simulink model "flc_ann_master"  (R2025a)
settings: Solver=ode23tb  StartTime=0.0  StopTime=2  FixedStep=1e-8  MaxStep=1e-5  RelTol=1e-4
values from neighbouring files (symbols this model uses):
  init_duty = 0.5    [params.m]    (also in sim_duties.m = init_duty_array(i))
  irr_final_1 = 1000    [sim_duties.m]
  irr_final_2 = 1000    [sim_duties.m]
  irr_final_3 = 1000    [sim_duties.m]
  irr_final_4 = 1000    [sim_duties.m]
  irr_final_5 = 1000    [sim_duties.m]
  irr_init_1 = 1000    [sim_duties.m]
  irr_init_2 = 1000    [sim_duties.m]
  irr_init_3 = 1000    [sim_duties.m]
  irr_init_4 = 1000    [sim_duties.m]
  irr_init_5 = 1000    [sim_duties.m]
  sample_time_FLC = 0.005    [params.m]    (also in sim_duties.m)
  sample_time_mv_avg = 1e-4    (= 0.0001)    [params.m]    (also in sim_duties.m)
  temp = 25    [params.m]    (also in sim_duties.m)
undefined symbols (not defined in the file or in its folder): DiscIntNeverNeededParam, t_step
libraries: neural x36, spsMosfetLib x5, spsSeriesRLCBranchLib x5, eeGeneralControl x3, spsCurrentMeasurementLib x2, spsDiodeLib x2, spsFirstOrderFilterLib x2, slpidlib x2, simulink x2, spsVoltageMeasurementLib x2, spsACVoltageSourceLib x1, spsAlphaBetaZerotodq0Lib x1
(part 2 of 2)

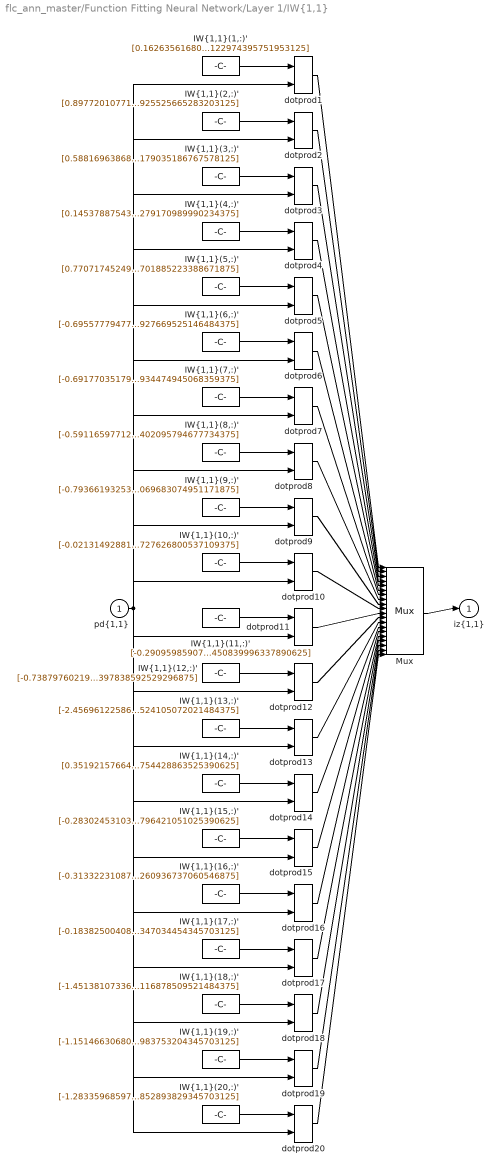
== system flc_ann_master/Function Fitting Neural Network/Layer 1/IW{1,1} ==
  "pd{1,1}" : Inport  PortDimensions=5
      mask Display: e = 0.06;c1 = [120 230 180]/255;c2 = ([120 230 180]+0)/(256+128);c3 = ([120 230 180]+128)/(256+128);patch([0 1 1 0],[0 0 1 1],c1);patch([0 1 1 1-e 1-e 0+e],[0 0 1 1-e 0+e 0+e],c2);patch([0 0 1 1-e 0+e 0+e],[0 1 1 1-e 1-e 0+e],c3);plot([0 1 1 0 0],[0 0 1 1 0]);
  "IW{1,1}(1,:)'" : Constant  Value=[0.1626356168023161130609111069134087301790714263916015625;1.014539472778073214698224546737037599086761474609375;1.99974778893698879045359717565588653087615966796875;0.2096339514215423971421614623977802693843841552734375;-5.6789966587194289360240873065777122974395751953125]
      mask Display: e = 0.06;c1 = [120 150 230]/255;c2 = ([120 150 230]+0)/383;c3 = ([120 150 230]+128)/383;patch([0 1 1 0],[0 0 1 1],c1);patch([0 1 1 1-e 1-e 0+e],[0 0 1 1-e 0+e 0+e],c2);patch([0 0 1 1-e 0+e 0+e],[0 1 1 1-e 1-e 0+e],c3);plot([0 1 1 0 0],[0 0 1 1 0]);disp('Weights');
  "IW{1,1}(10,:)'" : Constant  Value=[-0.0213149288150113642992256046682086889632046222686767578125;-0.568850920387156566704334181849844753742218017578125;1.371346571730940322453307089745067059993743896484375;1.577494106987263666752596691367216408252716064453125;-0.39484466016965702461760656660771928727626800537109375]
      mask Display: e = 0.06;c1 = [120 150 230]/255;c2 = ([120 150 230]+0)/383;c3 = ([120 150 230]+128)/383;patch([0 1 1 0],[0 0 1 1],c1);patch([0 1 1 1-e 1-e 0+e],[0 0 1 1-e 0+e 0+e],c2);patch([0 0 1 1-e 0+e 0+e],[0 1 1 1-e 1-e 0+e],c3);plot([0 1 1 0 0],[0 0 1 1 0]);disp('Weights');
  "IW{1,1}(11,:)'" : Constant  Value=[-0.29095985907524279934222022347967140376567840576171875;1.4011731136993168522764108274714089930057525634765625;1.1829639348115577046627322488347999751567840576171875;-5.07892395952207653664345343713648617267608642578125;2.99724620350438275551141487085260450839996337890625]
      mask Display: e = 0.06;c1 = [120 150 230]/255;c2 = ([120 150 230]+0)/383;c3 = ([120 150 230]+128)/383;patch([0 1 1 0],[0 0 1 1],c1);patch([0 1 1 1-e 1-e 0+e],[0 0 1 1-e 0+e 0+e],c2);patch([0 0 1 1-e 0+e 0+e],[0 1 1 1-e 1-e 0+e],c3);plot([0 1 1 0 0],[0 0 1 1 0]);disp('Weights');
  "IW{1,1}(12,:)'" : Constant  Value=[-0.7387976021984303809375660421210341155529022216796875;-1.0178618623283923749767154731671325862407684326171875;-0.1381009052088023880688893996193655766546726226806640625;0.59120561994734599498002580730826593935489654541015625;1.826460521302780914965069314348511397838592529296875]
      mask Display: e = 0.06;c1 = [120 150 230]/255;c2 = ([120 150 230]+0)/383;c3 = ([120 150 230]+128)/383;patch([0 1 1 0],[0 0 1 1],c1);patch([0 1 1 1-e 1-e 0+e],[0 0 1 1-e 0+e 0+e],c2);patch([0 0 1 1-e 0+e 0+e],[0 1 1 1-e 1-e 0+e],c3);plot([0 1 1 0 0],[0 0 1 1 0]);disp('Weights');
  "IW{1,1}(13,:)'" : Constant  Value=[-2.456961225860202713278113151318393647670745849609375;-0.5049152215026426748778476394363678991794586181640625;0.3922518923682936087260486601735465228557586669921875;0.6442280759956335867144616713630966842174530029296875;-0.51190556258231667552394128506421111524105072021484375]
      mask Display: e = 0.06;c1 = [120 150 230]/255;c2 = ([120 150 230]+0)/383;c3 = ([120 150 230]+128)/383;patch([0 1 1 0],[0 0 1 1],c1);patch([0 1 1 1-e 1-e 0+e],[0 0 1 1-e 0+e 0+e],c2);patch([0 0 1 1-e 0+e 0+e],[0 1 1 1-e 1-e 0+e],c3);plot([0 1 1 0 0],[0 0 1 1 0]);disp('Weights');
  "IW{1,1}(14,:)'" : Constant  Value=[0.351921576647878431298721579878474585711956024169921875;-2.29066783338849599971354109584353864192962646484375;-1.1972818394599020752622209329274483025074005126953125;1.964498776969650695178870591917075216770172119140625;2.312458865409122044098921833210624754428863525390625]
      mask Display: e = 0.06;c1 = [120 150 230]/255;c2 = ([120 150 230]+0)/383;c3 = ([120 150 230]+128)/383;patch([0 1 1 0],[0 0 1 1],c1);patch([0 1 1 1-e 1-e 0+e],[0 0 1 1-e 0+e 0+e],c2);patch([0 0 1 1-e 0+e 0+e],[0 1 1 1-e 1-e 0+e],c3);plot([0 1 1 0 0],[0 0 1 1 0]);disp('Weights');
  "IW{1,1}(15,:)'" : Constant  Value=[-0.283024531034079596114594323807978071272373199462890625;-0.64693582354276502055512310107587836682796478271484375;-1.91800918516954066461721595260314643383026123046875;-2.092225653502387761051295456127263605594635009765625;1.516845141309114186611850527697242796421051025390625]
      mask Display: e = 0.06;c1 = [120 150 230]/255;c2 = ([120 150 230]+0)/383;c3 = ([120 150 230]+128)/383;patch([0 1 1 0],[0 0 1 1],c1);patch([0 1 1 1-e 1-e 0+e],[0 0 1 1-e 0+e 0+e],c2);patch([0 0 1 1-e 0+e 0+e],[0 1 1 1-e 1-e 0+e],c3);plot([0 1 1 0 0],[0 0 1 1 0]);disp('Weights');
  "IW{1,1}(16,:)'" : Constant  Value=[-0.313322310879322218912790276590385474264621734619140625;2.774701737691696035170707546058110892772674560546875;-4.53633611923154145273429094231687486171722412109375;-0.65501382413655140357633399617043323814868927001953125;-0.9854404943783190429229534856858663260936737060546875]
      mask Display: e = 0.06;c1 = [120 150 230]/255;c2 = ([120 150 230]+0)/383;c3 = ([120 150 230]+128)/383;patch([0 1 1 0],[0 0 1 1],c1);patch([0 1 1 1-e 1-e 0+e],[0 0 1 1-e 0+e 0+e],c2);patch([0 0 1 1-e 0+e 0+e],[0 1 1 1-e 1-e 0+e],c3);plot([0 1 1 0 0],[0 0 1 1 0]);disp('Weights');
  "IW{1,1}(17,:)'" : Constant  Value=[-0.1838250040857035416674847283502458594739437103271484375;1.130320574163679037127394622075371444225311279296875;-1.213329860734431608904060340137220919132232666015625;-1.884962772921485285593234948464669287204742431640625;0.98188732582681570448812635731883347034454345703125]
      mask Display: e = 0.06;c1 = [120 150 230]/255;c2 = ([120 150 230]+0)/383;c3 = ([120 150 230]+128)/383;patch([0 1 1 0],[0 0 1 1],c1);patch([0 1 1 1-e 1-e 0+e],[0 0 1 1-e 0+e 0+e],c2);patch([0 0 1 1-e 0+e 0+e],[0 1 1 1-e 1-e 0+e],c3);plot([0 1 1 0 0],[0 0 1 1 0]);disp('Weights');
  "IW{1,1}(18,:)'" : Constant  Value=[-1.4513810733606338221335363414254970848560333251953125;2.008917038973344393326669887755997478961944580078125;1.3543511781589836484585021025850437581539154052734375;0.07174802344186757829813672060481621883809566497802734375;0.28193094730051215801580610786913894116878509521484375]
      mask Display: e = 0.06;c1 = [120 150 230]/255;c2 = ([120 150 230]+0)/383;c3 = ([120 150 230]+128)/383;patch([0 1 1 0],[0 0 1 1],c1);patch([0 1 1 1-e 1-e 0+e],[0 0 1 1-e 0+e 0+e],c2);patch([0 0 1 1-e 0+e 0+e],[0 1 1 1-e 1-e 0+e],c3);plot([0 1 1 0 0],[0 0 1 1 0]);disp('Weights');
  "IW{1,1}(19,:)'" : Constant  Value=[-1.1514663068085624342273831643979065120220184326171875;1.380766100437355259344940350274555385112762451171875;-0.448457718469357835555655356074566952884197235107421875;1.169745525191284940547120640985667705535888671875;1.352602327310475249788623841595835983753204345703125]
      mask Display: e = 0.06;c1 = [120 150 230]/255;c2 = ([120 150 230]+0)/383;c3 = ([120 150 230]+128)/383;patch([0 1 1 0],[0 0 1 1],c1);patch([0 1 1 1-e 1-e 0+e],[0 0 1 1-e 0+e 0+e],c2);patch([0 0 1 1-e 0+e 0+e],[0 1 1 1-e 1-e 0+e],c3);plot([0 1 1 0 0],[0 0 1 1 0]);disp('Weights');
  "IW{1,1}(2,:)'" : Constant  Value=[0.897720107718310789124416260165162384510040283203125;0.6045958291500983516897349545615725219249725341796875;1.7980406071958838776225775291095487773418426513671875;-4.24893179252118624589229511911980807781219482421875;-0.7416107529120250507759237734717316925525665283203125]
      mask Display: e = 0.06;c1 = [120 150 230]/255;c2 = ([120 150 230]+0)/383;c3 = ([120 150 230]+128)/383;patch([0 1 1 0],[0 0 1 1],c1);patch([0 1 1 1-e 1-e 0+e],[0 0 1 1-e 0+e 0+e],c2);patch([0 0 1 1-e 0+e 0+e],[0 1 1 1-e 1-e 0+e],c3);plot([0 1 1 0 0],[0 0 1 1 0]);disp('Weights');
  "IW{1,1}(20,:)'" : Constant  Value=[-1.28335968597945448976815896457992494106292724609375;-1.4230720872940150201202413882128894329071044921875;-1.383852677357449767470143342507071793079376220703125;-0.2359179865147377486156443637810298241674900054931640625;-0.201423945604798593222994895768351852893829345703125]
      mask Display: e = 0.06;c1 = [120 150 230]/255;c2 = ([120 150 230]+0)/383;c3 = ([120 150 230]+128)/383;patch([0 1 1 0],[0 0 1 1],c1);patch([0 1 1 1-e 1-e 0+e],[0 0 1 1-e 0+e 0+e],c2);patch([0 0 1 1-e 0+e 0+e],[0 1 1 1-e 1-e 0+e],c3);plot([0 1 1 0 0],[0 0 1 1 0]);disp('Weights');
  "IW{1,1}(3,:)'" : Constant  Value=[0.5881696386836756662574998699710704386234283447265625;-0.89580513472184242207418947145924903452396392822265625;-1.5454054003772699221741504516103304922580718994140625;0.955378626380716244881341481232084333896636962890625;1.1847012618567938080360590902273543179035186767578125]
      mask Display: e = 0.06;c1 = [120 150 230]/255;c2 = ([120 150 230]+0)/383;c3 = ([120 150 230]+128)/383;patch([0 1 1 0],[0 0 1 1],c1);patch([0 1 1 1-e 1-e 0+e],[0 0 1 1-e 0+e 0+e],c2);patch([0 0 1 1-e 0+e 0+e],[0 1 1 1-e 1-e 0+e],c3);plot([0 1 1 0 0],[0 0 1 1 0]);disp('Weights');
  "IW{1,1}(4,:)'" : Constant  Value=[0.1453788754354973511428994470406905747950077056884765625;1.6569375264883834386608896238612942397594451904296875;-3.56372497066039262136882825870998203754425048828125;-0.8353641157188942401035092188976705074310302734375;1.2124796973580609371623495462699793279170989990234375]
      mask Display: e = 0.06;c1 = [120 150 230]/255;c2 = ([120 150 230]+0)/383;c3 = ([120 150 230]+128)/383;patch([0 1 1 0],[0 0 1 1],c1);patch([0 1 1 1-e 1-e 0+e],[0 0 1 1-e 0+e 0+e],c2);patch([0 0 1 1-e 0+e 0+e],[0 1 1 1-e 1-e 0+e],c3);plot([0 1 1 0 0],[0 0 1 1 0]);disp('Weights');
  "IW{1,1}(5,:)'" : Constant  Value=[0.77071745249031808899786710753687657415866851806640625;0.3806567747078062335930326298694126307964324951171875;-1.1569156708901997543392781153670512139797210693359375;3.0882529402780907190617654123343527317047119140625;-0.462094404994892016258489775282214395701885223388671875]
      mask Display: e = 0.06;c1 = [120 150 230]/255;c2 = ([120 150 230]+0)/383;c3 = ([120 150 230]+128)/383;patch([0 1 1 0],[0 0 1 1],c1);patch([0 1 1 1-e 1-e 0+e],[0 0 1 1-e 0+e 0+e],c2);patch([0 0 1 1-e 0+e 0+e],[0 1 1 1-e 1-e 0+e],c3);plot([0 1 1 0 0],[0 0 1 1 0]);disp('Weights');
  "IW{1,1}(6,:)'" : Constant  Value=[-0.695577794775811497629547375254333019256591796875;-1.701146701078736445111871944391168653964996337890625;-2.050427426016556697874193559982813894748687744140625;1.811004933153217422159286797977983951568603515625;-0.49416975187174771999565336955129168927669525146484375]
      mask Display: e = 0.06;c1 = [120 150 230]/255;c2 = ([120 150 230]+0)/383;c3 = ([120 150 230]+128)/383;patch([0 1 1 0],[0 0 1 1],c1);patch([0 1 1 1-e 1-e 0+e],[0 0 1 1-e 0+e 0+e],c2);patch([0 0 1 1-e 0+e 0+e],[0 1 1 1-e 1-e 0+e],c3);plot([0 1 1 0 0],[0 0 1 1 0]);disp('Weights');
  "IW{1,1}(7,:)'" : Constant  Value=[-0.69177035179182977397971399113885127007961273193359375;-0.205470533347971773263651584784383885562419891357421875;1.7003040131834559200996181971277110278606414794921875;2.216435685343544292891238001175224781036376953125;1.451900915541782577378171481541357934474945068359375]
      mask Display: e = 0.06;c1 = [120 150 230]/255;c2 = ([120 150 230]+0)/383;c3 = ([120 150 230]+128)/383;patch([0 1 1 0],[0 0 1 1],c1);patch([0 1 1 1-e 1-e 0+e],[0 0 1 1-e 0+e 0+e],c2);patch([0 0 1 1-e 0+e 0+e],[0 1 1 1-e 1-e 0+e],c3);plot([0 1 1 0 0],[0 0 1 1 0]);disp('Weights');
  "IW{1,1}(8,:)'" : Constant  Value=[-0.5911659771272115282414461034932173788547515869140625;0.9796323024744155727461247806786559522151947021484375;-0.51058490400159783906275379194994457066059112548828125;1.178946871689596331833627118612639605998992919921875;1.0642800652213446621630055233254097402095794677734375]
      mask Display: e = 0.06;c1 = [120 150 230]/255;c2 = ([120 150 230]+0)/383;c3 = ([120 150 230]+128)/383;patch([0 1 1 0],[0 0 1 1],c1);patch([0 1 1 1-e 1-e 0+e],[0 0 1 1-e 0+e 0+e],c2);patch([0 0 1 1-e 0+e 0+e],[0 1 1 1-e 1-e 0+e],c3);plot([0 1 1 0 0],[0 0 1 1 0]);disp('Weights');
  "IW{1,1}(9,:)'" : Constant  Value=[-0.79366193253040240307427666266448795795440673828125;-2.096544268041097947019579805782996118068695068359375;1.5771254899472586519237893298850394785404205322265625;-0.648392743318678466124538317671976983547210693359375;-0.26633219699267030033951186851481907069683074951171875]
      mask Display: e = 0.06;c1 = [120 150 230]/255;c2 = ([120 150 230]+0)/383;c3 = ([120 150 230]+128)/383;patch([0 1 1 0],[0 0 1 1],c1);patch([0 1 1 1-e 1-e 0+e],[0 0 1 1-e 0+e 0+e],c2);patch([0 0 1 1-e 0+e 0+e],[0 1 1 1-e 1-e 0+e],c3);plot([0 1 1 0 0],[0 0 1 1 0]);disp('Weights');
  Mux : Mux  Inputs=20
      mask Display: e = 0.06;c1 = [120 150 230]/255;c2 = ([120 150 230]+0)/383;c3 = ([120 150 230]+128)/383;patch([0 1 1 0],[0 0 1 1],c1);patch([0 1 1 1-e 1-e 0+e],[0 0 1 1-e 0+e 0+e],c2);patch([0 0 1 1-e 0+e 0+e],[0 1 1 1-e 1-e 0+e],c3);plot([0 1 1 0 0],[0 0 1 1 0]);disp('Mux');
  dotprod{1..20} (20 alike) : neural/Weight Functions/dotprod
  "iz{1,1}" : Outport
      mask Display: e = 0.06;c1 = [120 230 180]/255;c2 = ([120 230 180]+0)/(256+128);c3 = ([120 230 180]+128)/(256+128);patch([0 1 1 0],[0 0 1 1],c1);patch([0 1 1 1-e 1-e 0+e],[0 0 1 1-e 0+e 0+e],c2);patch([0 0 1 1-e 0+e 0+e],[0 1 1 1-e 1-e 0+e],c3);plot([0 1 1 0 0],[0 0 1 1 0]);
  wires:
  "IW{1,1}(1,:)'"/1 -> dotprod1/1
  "pd{1,1}"/1 -> dotprod1/2, dotprod2/2, dotprod3/2, dotprod4/2, dotprod5/2, dotprod6/2, dotprod7/2, dotprod8/2, dotprod9/2, dotprod10/2, dotprod11/2, dotprod12/2, dotprod13/2, dotprod14/2, dotprod15/2, dotprod16/2, dotprod17/2, dotprod18/2, dotprod19/2, dotprod20/2
  dotprod1/1 -> Mux/1
  "IW{1,1}(2,:)'"/1 -> dotprod2/1
  dotprod2/1 -> Mux/2
  "IW{1,1}(3,:)'"/1 -> dotprod3/1
  dotprod3/1 -> Mux/3
  "IW{1,1}(4,:)'"/1 -> dotprod4/1
  dotprod4/1 -> Mux/4
  "IW{1,1}(5,:)'"/1 -> dotprod5/1
  dotprod5/1 -> Mux/5
  "IW{1,1}(6,:)'"/1 -> dotprod6/1
  dotprod6/1 -> Mux/6
  "IW{1,1}(7,:)'"/1 -> dotprod7/1
  dotprod7/1 -> Mux/7
  "IW{1,1}(8,:)'"/1 -> dotprod8/1
  dotprod8/1 -> Mux/8
  "IW{1,1}(9,:)'"/1 -> dotprod9/1
  dotprod9/1 -> Mux/9
  "IW{1,1}(10,:)'"/1 -> dotprod10/1
  dotprod10/1 -> Mux/10
  "IW{1,1}(11,:)'"/1 -> dotprod11/1
  dotprod11/1 -> Mux/11
  "IW{1,1}(12,:)'"/1 -> dotprod12/1
  dotprod12/1 -> Mux/12
  "IW{1,1}(13,:)'"/1 -> dotprod13/1
  dotprod13/1 -> Mux/13
  "IW{1,1}(14,:)'"/1 -> dotprod14/1
  dotprod14/1 -> Mux/14
  "IW{1,1}(15,:)'"/1 -> dotprod15/1
  dotprod15/1 -> Mux/15
  "IW{1,1}(16,:)'"/1 -> dotprod16/1
  dotprod16/1 -> Mux/16
  "IW{1,1}(17,:)'"/1 -> dotprod17/1
  dotprod17/1 -> Mux/17
  "IW{1,1}(18,:)'"/1 -> dotprod18/1
  dotprod18/1 -> Mux/18
  "IW{1,1}(19,:)'"/1 -> dotprod19/1
  dotprod19/1 -> Mux/19
  "IW{1,1}(20,:)'"/1 -> dotprod20/1
  dotprod20/1 -> Mux/20
  Mux/1 -> "iz{1,1}"/1

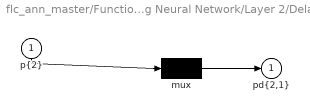
== system flc_ann_master/Function Fitting Neural Network/Layer 2/Delays 1 ==
  "p{2}" : Inport  PortDimensions=20
      mask Display: e = 0.06;c1 = [120 230 180]/255;c2 = ([120 230 180]+0)/(256+128);c3 = ([120 230 180]+128)/(256+128);patch([0 1 1 0],[0 0 1 1],c1);patch([0 1 1 1-e 1-e 0+e],[0 0 1 1-e 0+e 0+e],c2);patch([0 0 1 1-e 0+e 0+e],[0 1 1 1-e 1-e 0+e],c3);plot([0 1 1 0 0],[0 0 1 1 0]);
  mux : Mux  Inputs=1
      mask Display: e = 0.06;c1 = [120 150 230]/255;c2 = ([120 150 230]+0)/383;c3 = ([120 150 230]+128)/383;patch([0 1 1 0],[0 0 1 1],c1);patch([0 1 1 1-e 1-e 0+e],[0 0 1 1-e 0+e 0+e],c2);patch([0 0 1 1-e 0+e 0+e],[0 1 1 1-e 1-e 0+e],c3);plot([0 1 1 0 0],[0 0 1 1 0]);disp('Mux')
  "pd{2,1}" : Outport
      mask Display: e = 0.06;c1 = [120 230 180]/255;c2 = ([120 230 180]+0)/(256+128);c3 = ([120 230 180]+128)/(256+128);patch([0 1 1 0],[0 0 1 1],c1);patch([0 1 1 1-e 1-e 0+e],[0 0 1 1-e 0+e 0+e],c2);patch([0 0 1 1-e 0+e 0+e],[0 1 1 1-e 1-e 0+e],c3);plot([0 1 1 0 0],[0 0 1 1 0]);
  wires:
  "p{2}"/1 -> mux/1
  mux/1 -> "pd{2,1}"/1

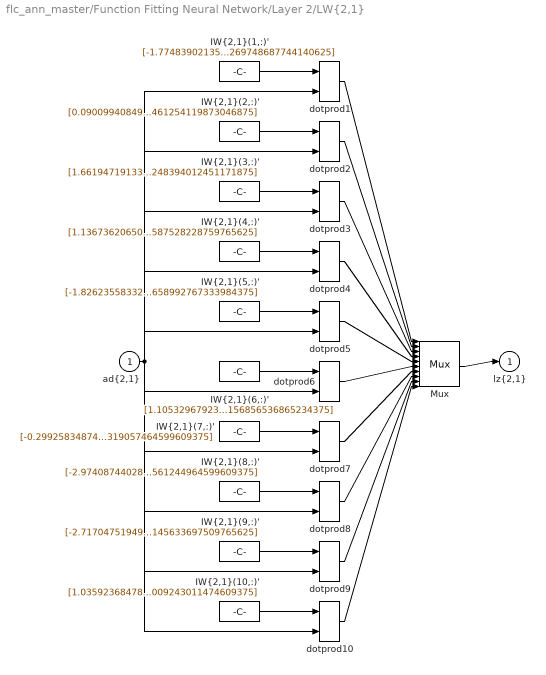
== system flc_ann_master/Function Fitting Neural Network/Layer 2/LW{2,1} ==
  "ad{2,1}" : Inport  PortDimensions=20
      mask Display: e = 0.06;c1 = [120 230 180]/255;c2 = ([120 230 180]+0)/(256+128);c3 = ([120 230 180]+128)/(256+128);patch([0 1 1 0],[0 0 1 1],c1);patch([0 1 1 1-e 1-e 0+e],[0 0 1 1-e 0+e 0+e],c2);patch([0 0 1 1-e 0+e 0+e],[0 1 1 1-e 1-e 0+e],c3);plot([0 1 1 0 0],[0 0 1 1 0]);
  "IW{2,1}(1,:)'" : Constant  Value=[-1.7748390213516829216899850507616065442562103271484375;-1.0851905161082211481726744750631041824817657470703125;0.0879655212133775565863658130183466710150241851806640625;-0.2427956672680668948061111223069019615650177001953125;-0.41620734711731188770755807126988656818866729736328125;0.1118016612279006116725810215939418412744998931884765625;0.175553249733231109264153246840578503906726837158203125;0.58816723003619753029624916962347924709320068359375;-0.71364399640571141159028911715722642838954925537109375;-0.358126071846602000992021430647582747042179107666015625;-1.557492327660729980465248445398174226284027099609375;-0.411557845238488206884852615985437296330928802490234375;0.162069140814274315065546261394047178328037261962890625;0.2018697442813035258790677062279428355395793914794921875;0.59143096942646966596157653839327394962310791015625;-2.6048171582415147184974557603709399700164794921875;0.1086056158994691822616829313119524158537387847900390625;0.1627455663637290828038572954028495587408542633056640625;-0.7658714525679306550642877482459880411624908447265625;-0.0115076427517147618362347571974169113673269748687744140625]
      mask Display: e = 0.06;c1 = [120 150 230]/255;c2 = ([120 150 230]+0)/383;c3 = ([120 150 230]+128)/383;patch([0 1 1 0],[0 0 1 1],c1);patch([0 1 1 1-e 1-e 0+e],[0 0 1 1-e 0+e 0+e],c2);patch([0 0 1 1-e 0+e 0+e],[0 1 1 1-e 1-e 0+e],c3);plot([0 1 1 0 0],[0 0 1 1 0]);disp('weights');
  "IW{2,1}(10,:)'" : Constant  Value=[1.0359236847871040598789704745286144316196441650390625;-0.9294544274639078285105142640531994402408599853515625;0.00110461130259771091177700697016916819848120212554931640625;0.2097605605665133765569407842122018337249755859375;0.04648220670897040829316892995848320424556732177734375;-0.50057924530877617730340034540859051048755645751953125;0.0269872595856186538176846312353518442250788211822509765625;0.46222712340660676577641652329475618898868560791015625;-0.00039030348449288487788777501918957568705081939697265625;0.0965990024143379699683720218672533519566059112548828125;-0.11705179672976806504181013224297203123569488525390625;-0.422539257683443025825908989645540714263916015625;0.008718879493650501244506045850357622839510440826416015625;0.6288058036628976221749098840518854558467864990234375;0.6861566586023701841412503199535422027111053466796875;-0.321104979890372899120620786561630666255950927734375;-0.054679911756703447611727142430027015507221221923828125;-0.241483457039892324136332035777741111814975738525390625;-0.220682281987896689035011377200135029852390289306640625;-0.317751911087980010162112876059836708009243011474609375]
      mask Display: e = 0.06;c1 = [120 150 230]/255;c2 = ([120 150 230]+0)/383;c3 = ([120 150 230]+128)/383;patch([0 1 1 0],[0 0 1 1],c1);patch([0 1 1 1-e 1-e 0+e],[0 0 1 1-e 0+e 0+e],c2);patch([0 0 1 1-e 0+e 0+e],[0 1 1 1-e 1-e 0+e],c3);plot([0 1 1 0 0],[0 0 1 1 0]);disp('weights');
  "IW{2,1}(2,:)'" : Constant  Value=[0.0900994084991108834525874726750771515071392059326171875;-0.42275002843330344859396063839085400104522705078125;0.41106945283283469194657300249673426151275634765625;-0.0328286555751075848075259955294313840568065643310546875;0.15938645575183851832434811512939631938934326171875;0.2281570675148948124100201084729633294045925140380859375;-0.611912607337229186299509819946251809597015380859375;-0.273033680250259924715550141627318225800991058349609375;0.63116445169487089827953241183422505855560302734375;0.1895748129025275063863631430649547837674617767333984375;-0.0060787486754775889308266556554372073151171207427978515625;-0.36171458411058232673696011261199600994586944580078125;0.283850684208339198999482277940842323005199432373046875;-0.2474918743750768868050471382957766763865947723388671875;-0.405811534579807620115587951659108512103557586669921875;-0.726834319771792802811205547186546027660369873046875;0.13110887519350733487755178430234082043170928955078125;-0.1730834090819354520451867074370966292917728424072265625;0.3800702386760799189602266778820194303989410400390625;0.61614772726251654244578048746916465461254119873046875]
      mask Display: e = 0.06;c1 = [120 150 230]/255;c2 = ([120 150 230]+0)/383;c3 = ([120 150 230]+128)/383;patch([0 1 1 0],[0 0 1 1],c1);patch([0 1 1 1-e 1-e 0+e],[0 0 1 1-e 0+e 0+e],c2);patch([0 0 1 1-e 0+e 0+e],[0 1 1 1-e 1-e 0+e],c3);plot([0 1 1 0 0],[0 0 1 1 0]);disp('weights');
  "IW{2,1}(3,:)'" : Constant  Value=[1.6619471913356724801502650734619237482547760009765625;0.80320888425067316074290602045948617160320281982421875;-0.42974621181859051777252034298726357519626617431640625;2.012260363216693992427508419496007263660430908203125;0.3829461937101334978450495327706448733806610107421875;0.2698697090464585723879054057761095464229583740234375;0.40440163734447154286755221619387157261371612548828125;0.30988402409611370824649156929808668792247772216796875;-0.12221027396480825533142677841169643215835094451904296875;0.1583872411342513164544953951917705126106739044189453125;-0.148870735175564650187851611917722038924694061279296875;0.20011297524720783602703022552304901182651519775390625;0.121527524159802169378963299095630645751953125;-0.584972673962948608306078313034959137439727783203125;-0.357330110653131693965178783400915563106536865234375;1.9207338833077221007528123664087615907192230224609375;-0.345078661045406576146632460222463123500347137451171875;-0.57567230834127591787563460457022301852703094482421875;0.40541761955673749628914492859621532261371612548828125;0.16505427245525694512906511590699665248394012451171875]
      mask Display: e = 0.06;c1 = [120 150 230]/255;c2 = ([120 150 230]+0)/383;c3 = ([120 150 230]+128)/383;patch([0 1 1 0],[0 0 1 1],c1);patch([0 1 1 1-e 1-e 0+e],[0 0 1 1-e 0+e 0+e],c2);patch([0 0 1 1-e 0+e 0+e],[0 1 1 1-e 1-e 0+e],c3);plot([0 1 1 0 0],[0 0 1 1 0]);disp('weights');
  "IW{2,1}(4,:)'" : Constant  Value=[1.1367362065094643863716328269219957292079925537109375;1.05867459455549717262101694359444081783294677734375;0.269367665032466785390852237469516694545745849609375;-0.073179360256906911263996562411193735897541046142578125;0.412632743924894296316807640323531813919544219970703125;-0.360755103613301597587081914753071032464504241943359375;-0.732153045567674354288101312704384326934814453125;0.39087665950779604262521615964942611753940582275390625;0.47868689941881392702072162137483246624469757080078125;0.456679921398484456318556112819351255893707275390625;-1.3053790239304652320839750245795585215091705322265625;-0.34771303026754873943815482562058605253696441650390625;-0.34198155256408380164856453120592050254344940185546875;-0.565998601620556929248095912043936550617218017578125;0.051267390610473494161336560637209913693368434906005859375;0.2554056580355370531520975418970920145511627197265625;0.7335557839287700776509382194490171968936920166015625;-0.1167629246669629472510365530979470349848270416259765625;0.291913105081559598463769589216099120676517486572265625;-0.28824398227018921403441709117032587528228759765625]
      mask Display: e = 0.06;c1 = [120 150 230]/255;c2 = ([120 150 230]+0)/383;c3 = ([120 150 230]+128)/383;patch([0 1 1 0],[0 0 1 1],c1);patch([0 1 1 1-e 1-e 0+e],[0 0 1 1-e 0+e 0+e],c2);patch([0 0 1 1-e 0+e 0+e],[0 1 1 1-e 1-e 0+e],c3);plot([0 1 1 0 0],[0 0 1 1 0]);disp('weights');
  "IW{2,1}(5,:)'" : Constant  Value=[-1.826235583329732126145472648204304277896881103515625;-0.69174878136150341756405168780474923551082611083984375;-0.393418788228750260227428725556819699704647064208984375;-1.0620556845446886828909782707341946661472320556640625;-0.00764801507747457816333014335441475850529968738555908203125;0.261514736239930767336403505396447144448757171630859375;0.258020686928107700897072618317906744778156280517578125;-0.5260764088624962919737981792422942817211151123046875;0.27723385747851636562444355149636976420879364013671875;-0.1805935486053139860107563663405016995966434478759765625;0.2123279740958931294247946652831160463392734527587890625;0.79799483294942497035862061238731257617473602294921875;-0.6787778804474893235010313219390809535980224609375;-0.381150475988623949064049156731925904750823974609375;-0.555774450499154415439306831103749573230743408203125;-1.70371814776133323476869918522424995899200439453125;0.017560874646031697510206726065007387660443782806396484375;0.1759351025154474168488150098710320889949798583984375;-0.324632070529664529257019012220553122460842132568359375;-0.094816521793870067735809925579815171658992767333984375]
      mask Display: e = 0.06;c1 = [120 150 230]/255;c2 = ([120 150 230]+0)/383;c3 = ([120 150 230]+128)/383;patch([0 1 1 0],[0 0 1 1],c1);patch([0 1 1 1-e 1-e 0+e],[0 0 1 1-e 0+e 0+e],c2);patch([0 0 1 1-e 0+e 0+e],[0 1 1 1-e 1-e 0+e],c3);plot([0 1 1 0 0],[0 0 1 1 0]);disp('weights');
  "IW{2,1}(6,:)'" : Constant  Value=[1.10532967923352298811323635163716971874237060546875;0.425508151839857740039718692059977911412715911865234375;0.2810528728220818006633408003835938870906829833984375;-1.02251042170248229723483746056444942951202392578125;-0.16754890745086481462777783235651440918445587158203125;-0.313762393223137425746216422339784912765026092529296875;-0.1109103102018910436132870245273807086050510406494140625;-0.66457990123790200431841412864741869270801544189453125;0.08575875291633709707195265536938677541911602020263671875;0.6382989440852282481131396707496605813503265380859375;-1.010472895895279332734162380802445113658905029296875;-0.52777310717398806527711485614418052136898040771484375;0.52201852859700947906418377897352911531925201416015625;-0.242402498080401762603486304215039126574993133544921875;-0.026944002098299064951181236438060295768082141876220703125;0.2360049966117288289257913902474683709442615509033203125;-0.2164248528020891182421792109380476176738739013671875;-0.3873600368042726671546915895305573940277099609375;-0.2342034900968595068082578336543519981205463409423828125;-0.159934535853247350445371921523474156856536865234375]
      mask Display: e = 0.06;c1 = [120 150 230]/255;c2 = ([120 150 230]+0)/383;c3 = ([120 150 230]+128)/383;patch([0 1 1 0],[0 0 1 1],c1);patch([0 1 1 1-e 1-e 0+e],[0 0 1 1-e 0+e 0+e],c2);patch([0 0 1 1-e 0+e 0+e],[0 1 1 1-e 1-e 0+e],c3);plot([0 1 1 0 0],[0 0 1 1 0]);disp('weights');
  "IW{2,1}(7,:)'" : Constant  Value=[-0.299258348746087754488343080083723179996013641357421875;-1.27059337710567366031000346993096172809600830078125;-0.258456223373940918719426917959935963153839111328125;-0.376115397441007193179984824382700026035308837890625;0.299919467564061736908342936658300459384918212890625;0.318543707591856684047115777502767741680145263671875;0.25651499705257829742066633116337470710277557373046875;0.50563208687369265437183685207855887711048126220703125;-0.60940614738906162539677779932389967143535614013671875;-0.36948148233138733420588550870888866484165191650390625;-1.36740465360285856633026924100704491138458251953125;0.429685486712592379365815986602683551609516143798828125;0.37131710337406287347761235650978051126003265380859375;-1.1453192166115402361725728042074479162693023681640625;0.404837609852881363803334124895627610385417938232421875;-1.1388077013808326487520616865367628633975982666015625;-0.17790024841783946829565365987946279346942901611328125;0.117369387771605715453659968261490575969219207763671875;0.07712176796942256384870262309050303883850574493408203125;0.003225440668542932376450238507459289394319057464599609375]
      mask Display: e = 0.06;c1 = [120 150 230]/255;c2 = ([120 150 230]+0)/383;c3 = ([120 150 230]+128)/383;patch([0 1 1 0],[0 0 1 1],c1);patch([0 1 1 1-e 1-e 0+e],[0 0 1 1-e 0+e 0+e],c2);patch([0 0 1 1-e 0+e 0+e],[0 1 1 1-e 1-e 0+e],c3);plot([0 1 1 0 0],[0 0 1 1 0]);disp('weights');
  "IW{2,1}(8,:)'" : Constant  Value=[-2.97408744028829463701413260423578321933746337890625;-2.876785291528384025383502375916577875614166259765625;0.12506364414988280220342176107806153595447540283203125;0.5651679803039140193021694358321838080883026123046875;-0.57501114888896187604672149973339401185512542724609375;-0.64481366233521442143938884328235872089862823486328125;0.77048773543512971695434998764540068805217742919921875;-1.0107102936770762102725029762950725853443145751953125;-1.2639583530190370286305778790847398340702056884765625;-1.4478457696729349901687555757234804332256317138671875;-2.272355300845458003777821431867778301239013671875;0.135036721393649694622496326701366342604160308837890625;-0.036644932654480717737488504326393012888729572296142578125;0.1296372248800210791319642567032133229076862335205078125;-0.1358589481148822775136153495623148046433925628662109375;-3.1920738899738125837757252156734466552734375;0.93156912343336395476711686569615267217159271240234375;1.026155999825197451258418368524871766567230224609375;-0.5264517650944380289246282700332812964916229248046875;-0.688068726739739844333598739467561244964599609375]
      mask Display: e = 0.06;c1 = [120 150 230]/255;c2 = ([120 150 230]+0)/383;c3 = ([120 150 230]+128)/383;patch([0 1 1 0],[0 0 1 1],c1);patch([0 1 1 1-e 1-e 0+e],[0 0 1 1-e 0+e 0+e],c2);patch([0 0 1 1-e 0+e 0+e],[0 1 1 1-e 1-e 0+e],c3);plot([0 1 1 0 0],[0 0 1 1 0]);disp('weights');
  "IW{2,1}(9,:)'" : Constant  Value=[-2.717047519493369645005031998152844607830047607421875;-1.029783861340809014706110247061587870121002197265625;0.40111551673782475102569833325105719268321990966796875;1.057182988890251973401745999581180512905120849609375;-1.282085603439926391189374044188298285007476806640625;-1.18363375361310030342565369210205972194671630859375;0.56123984129660076103363053334760479629039764404296875;-0.25804078977190225696602965399506501853466033935546875;0.45026381976948248730963086927658878266811370849609375;0.2380953861712696573160741309038712643086910247802734375;3.2238682544726344758601044304668903350830078125;0.64799075343608258936711763453786261379718780517578125;-0.76897165530605426919663614171440713107585906982421875;2.740085657251821071866970669361762702465057373046875;1.0819279282912488415746565806330181658267974853515625;-2.0819213739474147217833888134919106960296630859375;0.060860285046801632091728606610558927059173583984375;-0.4747051934088777347398035999503917992115020751953125;0.04554770531481140694030074200782109983265399932861328125;-0.633339694191582314175548162893392145633697509765625]
      mask Display: e = 0.06;c1 = [120 150 230]/255;c2 = ([120 150 230]+0)/383;c3 = ([120 150 230]+128)/383;patch([0 1 1 0],[0 0 1 1],c1);patch([0 1 1 1-e 1-e 0+e],[0 0 1 1-e 0+e 0+e],c2);patch([0 0 1 1-e 0+e 0+e],[0 1 1 1-e 1-e 0+e],c3);plot([0 1 1 0 0],[0 0 1 1 0]);disp('weights');
  Mux : Mux  Inputs=10
      mask Display: e = 0.06;c1 = [120 150 230]/255;c2 = ([120 150 230]+0)/383;c3 = ([120 150 230]+128)/383;patch([0 1 1 0],[0 0 1 1],c1);patch([0 1 1 1-e 1-e 0+e],[0 0 1 1-e 0+e 0+e],c2);patch([0 0 1 1-e 0+e 0+e],[0 1 1 1-e 1-e 0+e],c3);plot([0 1 1 0 0],[0 0 1 1 0]);disp('Mux');
  dotprod{1..10} (10 alike) : neural/Weight Functions/dotprod
  "lz{2,1}" : Outport
      mask Display: e = 0.06;c1 = [120 230 180]/255;c2 = ([120 230 180]+0)/(256+128);c3 = ([120 230 180]+128)/(256+128);patch([0 1 1 0],[0 0 1 1],c1);patch([0 1 1 1-e 1-e 0+e],[0 0 1 1-e 0+e 0+e],c2);patch([0 0 1 1-e 0+e 0+e],[0 1 1 1-e 1-e 0+e],c3);plot([0 1 1 0 0],[0 0 1 1 0]);
  wires:
  "IW{2,1}(1,:)'"/1 -> dotprod1/1
  "ad{2,1}"/1 -> dotprod1/2, dotprod2/2, dotprod3/2, dotprod4/2, dotprod5/2, dotprod6/2, dotprod7/2, dotprod8/2, dotprod9/2, dotprod10/2
  dotprod1/1 -> Mux/1
  "IW{2,1}(2,:)'"/1 -> dotprod2/1
  dotprod2/1 -> Mux/2
  "IW{2,1}(3,:)'"/1 -> dotprod3/1
  dotprod3/1 -> Mux/3
  "IW{2,1}(4,:)'"/1 -> dotprod4/1
  dotprod4/1 -> Mux/4
  "IW{2,1}(5,:)'"/1 -> dotprod5/1
  dotprod5/1 -> Mux/5
  "IW{2,1}(6,:)'"/1 -> dotprod6/1
  dotprod6/1 -> Mux/6
  "IW{2,1}(7,:)'"/1 -> dotprod7/1
  dotprod7/1 -> Mux/7
  "IW{2,1}(8,:)'"/1 -> dotprod8/1
  dotprod8/1 -> Mux/8
  "IW{2,1}(9,:)'"/1 -> dotprod9/1
  dotprod9/1 -> Mux/9
  "IW{2,1}(10,:)'"/1 -> dotprod10/1
  dotprod10/1 -> Mux/10
  Mux/1 -> "lz{2,1}"/1

== system flc_ann_master/Function Fitting Neural Network/Layer 3/Delays 1 ==
  "p{3}" : Inport  PortDimensions=10
      mask Display: e = 0.06;c1 = [120 230 180]/255;c2 = ([120 230 180]+0)/(256+128);c3 = ([120 230 180]+128)/(256+128);patch([0 1 1 0],[0 0 1 1],c1);patch([0 1 1 1-e 1-e 0+e],[0 0 1 1-e 0+e 0+e],c2);patch([0 0 1 1-e 0+e 0+e],[0 1 1 1-e 1-e 0+e],c3);plot([0 1 1 0 0],[0 0 1 1 0]);
  mux : Mux  Inputs=1
      mask Display: e = 0.06;c1 = [120 150 230]/255;c2 = ([120 150 230]+0)/383;c3 = ([120 150 230]+128)/383;patch([0 1 1 0],[0 0 1 1],c1);patch([0 1 1 1-e 1-e 0+e],[0 0 1 1-e 0+e 0+e],c2);patch([0 0 1 1-e 0+e 0+e],[0 1 1 1-e 1-e 0+e],c3);plot([0 1 1 0 0],[0 0 1 1 0]);disp('Mux')
  "pd{3,2}" : Outport
      mask Display: e = 0.06;c1 = [120 230 180]/255;c2 = ([120 230 180]+0)/(256+128);c3 = ([120 230 180]+128)/(256+128);patch([0 1 1 0],[0 0 1 1],c1);patch([0 1 1 1-e 1-e 0+e],[0 0 1 1-e 0+e 0+e],c2);patch([0 0 1 1-e 0+e 0+e],[0 1 1 1-e 1-e 0+e],c3);plot([0 1 1 0 0],[0 0 1 1 0]);
  wires:
  "p{3}"/1 -> mux/1
  mux/1 -> "pd{3,2}"/1

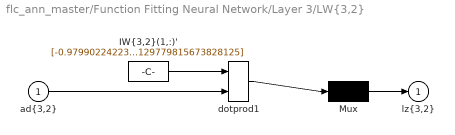
== system flc_ann_master/Function Fitting Neural Network/Layer 3/LW{3,2} ==
  "ad{3,2}" : Inport  PortDimensions=10
      mask Display: e = 0.06;c1 = [120 230 180]/255;c2 = ([120 230 180]+0)/(256+128);c3 = ([120 230 180]+128)/(256+128);patch([0 1 1 0],[0 0 1 1],c1);patch([0 1 1 1-e 1-e 0+e],[0 0 1 1-e 0+e 0+e],c2);patch([0 0 1 1-e 0+e 0+e],[0 1 1 1-e 1-e 0+e],c3);plot([0 1 1 0 0],[0 0 1 1 0]);
  "IW{3,2}(1,:)'" : Constant  Value=[-0.97990224223300737005359906106605194509029388427734375;-0.07055755405620507680897190994073753245174884796142578125;-1.060138289445408776856538679567165672779083251953125;0.222046496293034412161659929552115499973297119140625;-0.79264977853578211242080442389124073088169097900390625;0.046452936551062244674437096136898617260158061981201171875;0.416392592205831635343571406338014639914035797119140625;0.92623821662796412823581704287789762020111083984375;0.53942788782461537078205537909525446593761444091796875;-0.9006049682790930877018809042056091129779815673828125]
      mask Display: e = 0.06;c1 = [120 150 230]/255;c2 = ([120 150 230]+0)/383;c3 = ([120 150 230]+128)/383;patch([0 1 1 0],[0 0 1 1],c1);patch([0 1 1 1-e 1-e 0+e],[0 0 1 1-e 0+e 0+e],c2);patch([0 0 1 1-e 0+e 0+e],[0 1 1 1-e 1-e 0+e],c3);plot([0 1 1 0 0],[0 0 1 1 0]);disp('weights');
  Mux : Mux  Inputs=1
      mask Display: e = 0.06;c1 = [120 150 230]/255;c2 = ([120 150 230]+0)/383;c3 = ([120 150 230]+128)/383;patch([0 1 1 0],[0 0 1 1],c1);patch([0 1 1 1-e 1-e 0+e],[0 0 1 1-e 0+e 0+e],c2);patch([0 0 1 1-e 0+e 0+e],[0 1 1 1-e 1-e 0+e],c3);plot([0 1 1 0 0],[0 0 1 1 0]);disp('Mux');
  dotprod1 : neural/Weight Functions/dotprod
  "lz{3,2}" : Outport
      mask Display: e = 0.06;c1 = [120 230 180]/255;c2 = ([120 230 180]+0)/(256+128);c3 = ([120 230 180]+128)/(256+128);patch([0 1 1 0],[0 0 1 1],c1);patch([0 1 1 1-e 1-e 0+e],[0 0 1 1-e 0+e 0+e],c2);patch([0 0 1 1-e 0+e 0+e],[0 1 1 1-e 1-e 0+e],c3);plot([0 1 1 0 0],[0 0 1 1 0]);
  wires:
  "IW{3,2}(1,:)'"/1 -> dotprod1/1
  "ad{3,2}"/1 -> dotprod1/2
  dotprod1/1 -> Mux/1
  Mux/1 -> "lz{3,2}"/1

== matlab function flc_ann_master/MATLAB Function ==
  data: G1 input; G_sorted output; G2 input; G3 input; G4 input; G5 input
function G_sorted = fcn(G1, G2, G3, G4, G5)
    % Bundle inputs into an array and sort descending
    G_array = [G1, G2, G3, G4, G5];
    G_sorted = sort(G_array, 'descend');
end
